simulink model "worldbased"  (R2021a)
settings: Solver=VariableStepAuto  StartTime=0.0  StopTime=60  RelTol=1e-3
libraries: pid_lib x4, mpclib x1, aerolibfltsims x1
settings Model: Creator=ZumoArthicha  LastModifiedBy=ZumoArthicha

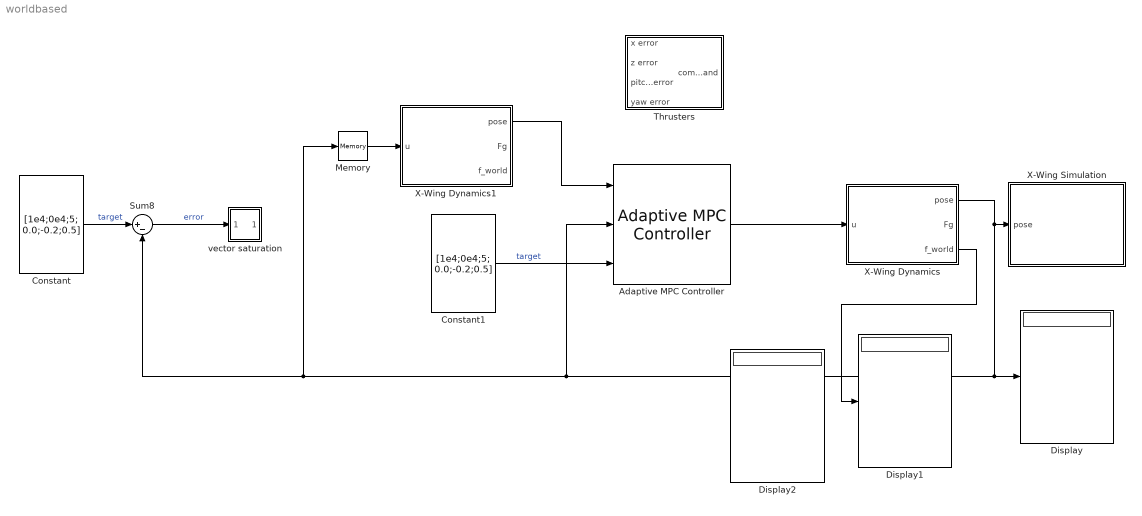
== system worldbased ==
  Adaptive MPC Controller : mpclib/Adaptive MPC Controller  SCDEnableBlockLinearizationSpecification=on  x0=[0;0;0;0;0;0]  enable_value=0  updateMPCinCallerWorkspace=on  md_inport=off  mv_inport=off  uref_inport=off  return_cost=off  return_mvseq=off  return_qpstatus=off  return_xseq=off  return_state=off  return_ovseq=off  state_inport=off  isltv_plant=off  umin_inport=off  umax_inport=off  ymin_inport=off  ymax_inport=off  cc_inport=off  ywt_inport=off  uwt_inport=off  duwt_inport=off  rhoeps_inport=off  pm_inport=off  MaximumP=10  HorizonChoice=FixedHorizon  BlockDataType=double  SampleTimeInherited=off  switch_inport=off
  Constant : Constant  Value=[1e4;0e4;5; 0.0;-0.2;0.5]  VectorParams1D=off
  Constant1 : Constant  Value=[1e4;0e4;5; 0.0;-0.2;0.5]  VectorParams1D=off
  Display : Display
  Display1 : Display
  Display2 : Display
  Memory : Memory
  Sum8 : Sum  Inputs=|+-
  Thrusters : Subsystem
      mask Display: image(imread("pictures/thrusters.PNG"))
  X-Wing Dynamics : Subsystem
      mask Display: image(imread("pictures/simplified_model.png"))
  X-Wing Dynamics1 : Subsystem
      mask Display: image(imread("pictures/simplified_model.png"))
  X-Wing Simulation : Subsystem
      mask Display: image(imread("pictures/simulation.PNG"))
  vector saturation : Subsystem
  wires:
  X-Wing Dynamics/1(pose) -> Display/1, Adaptive MPC Controller/2, Memory/1, Sum8/2, X-Wing Simulation/1(pose)
  Constant/1 -> Sum8/1  "target"
  Sum8/1 -> vector saturation/1(Input)  "error"
  X-Wing Dynamics/3(f_world) -> Display1/1
  Adaptive MPC Controller/1 -> X-Wing Dynamics/1(u)
  Constant1/1 -> Adaptive MPC Controller/3  "target"
  X-Wing Dynamics1/1(pose) -> Adaptive MPC Controller/1
  Memory/1 -> X-Wing Dynamics1/1(u)

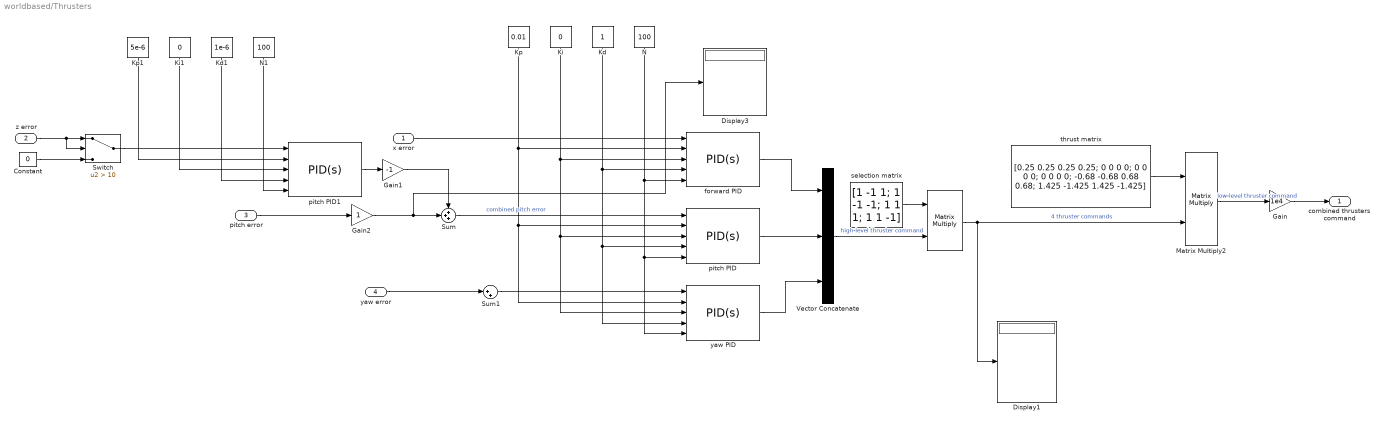
== system worldbased/Thrusters ==
  x error : Inport
  z error : Inport  Port=2
  pitch error : Inport  Port=3
  yaw error : Inport  Port=4
  "  " : Product  Multiplication=Matrix(*)
  Constant : Constant  Value=0
  Display1 : Display
  Display3 : Display
  Gain : Gain  Gain=1e4
  Gain1 : Gain  Gain=-1
  Gain2 : Gain
  Kd : Constant
  Kd1 : Constant  Value=1e-6
  Ki : Constant  Value=0
  Ki1 : Constant  Value=0
  Kp : Constant  Value=0.01
  Kp1 : Constant  Value=5e-6
  Matrix Multiply2 : Product  Multiplication=Matrix(*)
  N : Constant  Value=100
  N1 : Constant  Value=100
  Sum : Sum  Inputs=+++
  Sum1 : Sum  Inputs=|++
  Switch : Switch  Criteria=u2 > Threshold  Threshold=10
  Vector Concatenate : Concatenate  NumInputs=3
  forward PID : pid_lib/PID Controller  Controller=PID  Form=Parallel  TimeDomain=Continuous-time  UseExternalTs=off  SampleTime=-1  IntegratorMethod=Forward Euler  FilterMethod=Forward Euler  ControllerParametersSource=external  P=0.01  I=0  D=1  UseFilter=on  N=100  TunerSelectOption=Transfer Function Based (PID Tuner App)  InitialConditionSource=internal  InitialConditionForIntegrator=0  InitialConditionForFilter=0  DifferentiatorICPrevScaledInput=0  ExternalReset=none  TrackingMode=off  Kt=1  LimitOutput=off  SatLimitsSource=internal  UpperSaturationLimit=inf  LowerSaturationLimit=-inf  LinearizeAsGain=on  AntiWindupMode=none  Kb=1  POutMin=[]  POutMax=[]  IOutMin=[]  IOutMax=[]  DOutMin=[]  DOutMax=[]  NOutMin=[]  NOutMax=[]  SumOutMin=[]  SumOutMax=[]  SaturationOutMin=[]  SaturationOutMax=[]  PParamMin=[]  PParamMax=[]  IParamMin=[]  IParamMax=[]  DParamMin=[]  DParamMax=[]  NParamMin=[]  NParamMax=[]  KbParamMin=[]  KbParamMax=[]  KtParamMin=[]  KtParamMax=[]  KbOutMin=[]  KbOutMax=[]  KtOutMin=[]  KtOutMax=[]  IntegratorOutMin=[]  IntegratorOutMax=[]  FilterOutMin=[]  FilterOutMax=[]  SumI1OutMin=[]  SumI1OutMax=[]  SumI2OutMin=[]  SumI2OutMax=[]  SumI3OutMin=[]  SumI3OutMax=[]  SumI4OutMin=[]  SumI4OutMax=[]  SumDOutMin=[]  SumDOutMax=[]  DifferentiatorOutMin=[]  DifferentiatorOutMax=[]  FilterDiffOutCoefMin=[]  FilterDiffOutCoefMax=[]  ReciprocalOutMin=[]  ReciprocalOutMax=[]  SumDenOutMin=[]  SumDenOutMax=[]  SumNumOutMin=[]  SumNumOutMax=[]  DivideOutMin=[]  DivideOutMax=[]  UdiffTsProdOutMin=[]  UdiffTsProdOutMax=[]  NTsProdOutMin=[]  NTsProdOutMax=[]  UintegralTsProdOutMin=[]  UintegralTsProdOutMax=[]  UngainTsProdOutMin=[]  UngainTsProdOutMax=[]  IntegratorContinuousStateAttributes=''  IntegratorStateMustResolveToSignalObject=off  IntegratorRTWStateStorageClass=Auto  FilterContinuousStateAttributes=''  FilterStateMustResolveToSignalObject=off  FilterRTWStateStorageClass=Auto  ParallelPVariant=ExternalParameters  IdealPVariant=Disabled  IVariant=ExternalParameters  DVariant=ExternalParameters  IntegratorVariant=Continuous  SatVariant=Disabled  AWVariant=Passthrough  PCopyVariant=Disabled  TRVariant=Disabled  FdbkBlocksVariant=Forward  IdealPFdbkVariant=Disabled  SatFdbkVariant=Disabled  DerivativeFilterVariant=ContFilter  NVariant=ExternalParameters  NCopyVariant=Disabled  FilterICVariant=InternalICsFilter  IntegratorICVariant=InternalICs  ExternalResetVariant=Disabled  TRSumVariant=Passthrough  SumFdbkVariant=Disabled  SumVariant=Sum_PID  TsampFilterVariant=InternalTs  TsampNgainVariant=Passthrough  TsampIntegralVariant=Passthrough  ExternalSaturationOutDataTypeStr=Inherit: Same as second input
  pitch PID : pid_lib/PID Controller  Controller=PID  Form=Parallel  TimeDomain=Continuous-time  UseExternalTs=off  SampleTime=-1  IntegratorMethod=Forward Euler  FilterMethod=Forward Euler  ControllerParametersSource=external  P=0.01  I=0  D=1  UseFilter=on  N=100  TunerSelectOption=Transfer Function Based (PID Tuner App)  InitialConditionSource=internal  InitialConditionForIntegrator=0  InitialConditionForFilter=0  DifferentiatorICPrevScaledInput=0  ExternalReset=none  TrackingMode=off  Kt=1  LimitOutput=off  SatLimitsSource=internal  UpperSaturationLimit=inf  LowerSaturationLimit=-inf  LinearizeAsGain=on  AntiWindupMode=none  Kb=1  POutMin=[]  POutMax=[]  IOutMin=[]  IOutMax=[]  DOutMin=[]  DOutMax=[]  NOutMin=[]  NOutMax=[]  SumOutMin=[]  SumOutMax=[]  SaturationOutMin=[]  SaturationOutMax=[]  PParamMin=[]  PParamMax=[]  IParamMin=[]  IParamMax=[]  DParamMin=[]  DParamMax=[]  NParamMin=[]  NParamMax=[]  KbParamMin=[]  KbParamMax=[]  KtParamMin=[]  KtParamMax=[]  KbOutMin=[]  KbOutMax=[]  KtOutMin=[]  KtOutMax=[]  IntegratorOutMin=[]  IntegratorOutMax=[]  FilterOutMin=[]  FilterOutMax=[]  SumI1OutMin=[]  SumI1OutMax=[]  SumI2OutMin=[]  SumI2OutMax=[]  SumI3OutMin=[]  SumI3OutMax=[]  SumI4OutMin=[]  SumI4OutMax=[]  SumDOutMin=[]  SumDOutMax=[]  DifferentiatorOutMin=[]  DifferentiatorOutMax=[]  FilterDiffOutCoefMin=[]  FilterDiffOutCoefMax=[]  ReciprocalOutMin=[]  ReciprocalOutMax=[]  SumDenOutMin=[]  SumDenOutMax=[]  SumNumOutMin=[]  SumNumOutMax=[]  DivideOutMin=[]  DivideOutMax=[]  UdiffTsProdOutMin=[]  UdiffTsProdOutMax=[]  NTsProdOutMin=[]  NTsProdOutMax=[]  UintegralTsProdOutMin=[]  UintegralTsProdOutMax=[]  UngainTsProdOutMin=[]  UngainTsProdOutMax=[]  IntegratorContinuousStateAttributes=''  IntegratorStateMustResolveToSignalObject=off  IntegratorRTWStateStorageClass=Auto  FilterContinuousStateAttributes=''  FilterStateMustResolveToSignalObject=off  FilterRTWStateStorageClass=Auto  ParallelPVariant=ExternalParameters  IdealPVariant=Disabled  IVariant=ExternalParameters  DVariant=ExternalParameters  IntegratorVariant=Continuous  SatVariant=Disabled  AWVariant=Passthrough  PCopyVariant=Disabled  TRVariant=Disabled  FdbkBlocksVariant=Forward  IdealPFdbkVariant=Disabled  SatFdbkVariant=Disabled  DerivativeFilterVariant=ContFilter  NVariant=ExternalParameters  NCopyVariant=Disabled  FilterICVariant=InternalICsFilter  IntegratorICVariant=InternalICs  ExternalResetVariant=Disabled  TRSumVariant=Passthrough  SumFdbkVariant=Disabled  SumVariant=Sum_PID  TsampFilterVariant=InternalTs  TsampNgainVariant=Passthrough  TsampIntegralVariant=Passthrough  ExternalSaturationOutDataTypeStr=Inherit: Same as second input
  pitch PID1 : pid_lib/PID Controller  Controller=PID  Form=Parallel  TimeDomain=Continuous-time  UseExternalTs=off  SampleTime=-1  IntegratorMethod=Forward Euler  FilterMethod=Forward Euler  ControllerParametersSource=external  P=0.01  I=0  D=1  UseFilter=on  N=100  TunerSelectOption=Transfer Function Based (PID Tuner App)  InitialConditionSource=internal  InitialConditionForIntegrator=0  InitialConditionForFilter=0  DifferentiatorICPrevScaledInput=0  ExternalReset=none  TrackingMode=off  Kt=1  LimitOutput=off  SatLimitsSource=internal  UpperSaturationLimit=inf  LowerSaturationLimit=-inf  LinearizeAsGain=on  AntiWindupMode=none  Kb=1  POutMin=[]  POutMax=[]  IOutMin=[]  IOutMax=[]  DOutMin=[]  DOutMax=[]  NOutMin=[]  NOutMax=[]  SumOutMin=[]  SumOutMax=[]  SaturationOutMin=[]  SaturationOutMax=[]  PParamMin=[]  PParamMax=[]  IParamMin=[]  IParamMax=[]  DParamMin=[]  DParamMax=[]  NParamMin=[]  NParamMax=[]  KbParamMin=[]  KbParamMax=[]  KtParamMin=[]  KtParamMax=[]  KbOutMin=[]  KbOutMax=[]  KtOutMin=[]  KtOutMax=[]  IntegratorOutMin=[]  IntegratorOutMax=[]  FilterOutMin=[]  FilterOutMax=[]  SumI1OutMin=[]  SumI1OutMax=[]  SumI2OutMin=[]  SumI2OutMax=[]  SumI3OutMin=[]  SumI3OutMax=[]  SumI4OutMin=[]  SumI4OutMax=[]  SumDOutMin=[]  SumDOutMax=[]  DifferentiatorOutMin=[]  DifferentiatorOutMax=[]  FilterDiffOutCoefMin=[]  FilterDiffOutCoefMax=[]  ReciprocalOutMin=[]  ReciprocalOutMax=[]  SumDenOutMin=[]  SumDenOutMax=[]  SumNumOutMin=[]  SumNumOutMax=[]  DivideOutMin=[]  DivideOutMax=[]  UdiffTsProdOutMin=[]  UdiffTsProdOutMax=[]  NTsProdOutMin=[]  NTsProdOutMax=[]  UintegralTsProdOutMin=[]  UintegralTsProdOutMax=[]  UngainTsProdOutMin=[]  UngainTsProdOutMax=[]  IntegratorContinuousStateAttributes=''  IntegratorStateMustResolveToSignalObject=off  IntegratorRTWStateStorageClass=Auto  FilterContinuousStateAttributes=''  FilterStateMustResolveToSignalObject=off  FilterRTWStateStorageClass=Auto  ParallelPVariant=ExternalParameters  IdealPVariant=Disabled  IVariant=ExternalParameters  DVariant=ExternalParameters  IntegratorVariant=Continuous  SatVariant=Disabled  AWVariant=Passthrough  PCopyVariant=Disabled  TRVariant=Disabled  FdbkBlocksVariant=Forward  IdealPFdbkVariant=Disabled  SatFdbkVariant=Disabled  DerivativeFilterVariant=ContFilter  NVariant=ExternalParameters  NCopyVariant=Disabled  FilterICVariant=InternalICsFilter  IntegratorICVariant=InternalICs  ExternalResetVariant=Disabled  TRSumVariant=Passthrough  SumFdbkVariant=Disabled  SumVariant=Sum_PID  TsampFilterVariant=InternalTs  TsampNgainVariant=Passthrough  TsampIntegralVariant=Passthrough  ExternalSaturationOutDataTypeStr=Inherit: Same as second input
  selection matrix : Constant  Value=[1 -1 1; 1 -1 -1; 1 1 1; 1 1 -1]  VectorParams1D=off
  thrust matrix : Constant  Value=[0.25 0.25 0.25 0.25; 0 0 0 0; 0 0 0 0; 0 0 0 0; -0.68 -0.68 0.68 0.68; 1.425 -1.425 1.425 -1.425]  VectorParams1D=off
  yaw PID : pid_lib/PID Controller  Controller=PID  Form=Parallel  TimeDomain=Continuous-time  UseExternalTs=off  SampleTime=-1  IntegratorMethod=Forward Euler  FilterMethod=Forward Euler  ControllerParametersSource=external  P=0.01  I=0  D=1  UseFilter=on  N=100  TunerSelectOption=Transfer Function Based (PID Tuner App)  InitialConditionSource=internal  InitialConditionForIntegrator=0  InitialConditionForFilter=0  DifferentiatorICPrevScaledInput=0  ExternalReset=none  TrackingMode=off  Kt=1  LimitOutput=off  SatLimitsSource=internal  UpperSaturationLimit=inf  LowerSaturationLimit=-inf  LinearizeAsGain=on  AntiWindupMode=none  Kb=1  POutMin=[]  POutMax=[]  IOutMin=[]  IOutMax=[]  DOutMin=[]  DOutMax=[]  NOutMin=[]  NOutMax=[]  SumOutMin=[]  SumOutMax=[]  SaturationOutMin=[]  SaturationOutMax=[]  PParamMin=[]  PParamMax=[]  IParamMin=[]  IParamMax=[]  DParamMin=[]  DParamMax=[]  NParamMin=[]  NParamMax=[]  KbParamMin=[]  KbParamMax=[]  KtParamMin=[]  KtParamMax=[]  KbOutMin=[]  KbOutMax=[]  KtOutMin=[]  KtOutMax=[]  IntegratorOutMin=[]  IntegratorOutMax=[]  FilterOutMin=[]  FilterOutMax=[]  SumI1OutMin=[]  SumI1OutMax=[]  SumI2OutMin=[]  SumI2OutMax=[]  SumI3OutMin=[]  SumI3OutMax=[]  SumI4OutMin=[]  SumI4OutMax=[]  SumDOutMin=[]  SumDOutMax=[]  DifferentiatorOutMin=[]  DifferentiatorOutMax=[]  FilterDiffOutCoefMin=[]  FilterDiffOutCoefMax=[]  ReciprocalOutMin=[]  ReciprocalOutMax=[]  SumDenOutMin=[]  SumDenOutMax=[]  SumNumOutMin=[]  SumNumOutMax=[]  DivideOutMin=[]  DivideOutMax=[]  UdiffTsProdOutMin=[]  UdiffTsProdOutMax=[]  NTsProdOutMin=[]  NTsProdOutMax=[]  UintegralTsProdOutMin=[]  UintegralTsProdOutMax=[]  UngainTsProdOutMin=[]  UngainTsProdOutMax=[]  IntegratorContinuousStateAttributes=''  IntegratorStateMustResolveToSignalObject=off  IntegratorRTWStateStorageClass=Auto  FilterContinuousStateAttributes=''  FilterStateMustResolveToSignalObject=off  FilterRTWStateStorageClass=Auto  ParallelPVariant=ExternalParameters  IdealPVariant=Disabled  IVariant=ExternalParameters  DVariant=ExternalParameters  IntegratorVariant=Continuous  SatVariant=Disabled  AWVariant=Passthrough  PCopyVariant=Disabled  TRVariant=Disabled  FdbkBlocksVariant=Forward  IdealPFdbkVariant=Disabled  SatFdbkVariant=Disabled  DerivativeFilterVariant=ContFilter  NVariant=ExternalParameters  NCopyVariant=Disabled  FilterICVariant=InternalICsFilter  IntegratorICVariant=InternalICs  ExternalResetVariant=Disabled  TRSumVariant=Passthrough  SumFdbkVariant=Disabled  SumVariant=Sum_PID  TsampFilterVariant=InternalTs  TsampNgainVariant=Passthrough  TsampIntegralVariant=Passthrough  ExternalSaturationOutDataTypeStr=Inherit: Same as second input
  combined thrusters command : Outport  PortDimensions=6
  wires:
  N/1 -> yaw PID/5, pitch PID/5, forward PID/5
  Kd/1 -> pitch PID/4, yaw PID/4, forward PID/4
  Ki/1 -> yaw PID/3, pitch PID/3, forward PID/3
  Kp/1 -> pitch PID/2, yaw PID/2, forward PID/2
  yaw PID/1 -> Vector Concatenate/3
  x error/1 -> forward PID/1
  selection matrix/1 -> "  "/1
  Gain/1 -> combined thrusters command/1
  Matrix Multiply2/1 -> Gain/1  "low-level thruster command"
  thrust matrix/1 -> Matrix Multiply2/1
  Vector Concatenate/1 -> "  "/2  "high-level thruster command"
  "  "/1 -> Display1/1, Matrix Multiply2/2  "4 thruster commands"
  pitch PID1/1 -> Gain1/1
  Kp1/1 -> pitch PID1/2
  Ki1/1 -> pitch PID1/3
  Kd1/1 -> pitch PID1/4
  N1/1 -> pitch PID1/5
  Constant/1 -> Switch/3
  Switch/1 -> pitch PID1/1
  Sum/1 -> pitch PID/1  "combined pitch error"
  z error/1 -> Switch/2, Switch/1
  Gain2/1 -> Display3/1, Sum/2
  Sum1/1 -> yaw PID/1
  pitch PID/1 -> Vector Concatenate/2
  forward PID/1 -> Vector Concatenate/1
  pitch error/1 -> Gain2/1
  Gain1/1 -> Sum/1
  yaw error/1 -> Sum1/1

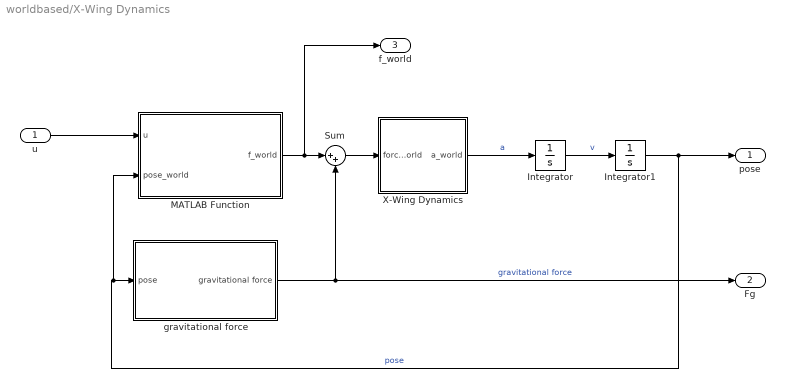
== system worldbased/X-Wing Dynamics ==
  u : Inport
  Integrator : Integrator  InitialCondition=[0;0;0;0;0;0]
  Integrator1 : Integrator  InitialCondition=[0;0;0;0;0;0]
  MATLAB Function : MATLAB Function  TreatAsAtomicUnit=on
  Sum : Sum  Inputs=|++
  X-Wing Dynamics : MATLAB Function  TreatAsAtomicUnit=on
  gravitational force : Subsystem
      mask Display: image(imread("pictures/gravitational_force.PNG"))
  pose : Outport
  Fg : Outport  Port=2
  f_world : Outport  Port=3
  wires:
  gravitational force/1(gravitational force) -> Fg/1, Sum/2  "gravitational force"
  Integrator/1 -> Integrator1/1  "v"
  Sum/1 -> X-Wing Dynamics/1(force_world)
  X-Wing Dynamics/1(a_world) -> Integrator/1  "a"
  Integrator1/1 -> pose/1, MATLAB Function/2(pose_world), gravitational force/1(pose)  "pose"
  u/1 -> MATLAB Function/1(u)
  MATLAB Function/1(f_world) -> f_world/1, Sum/1

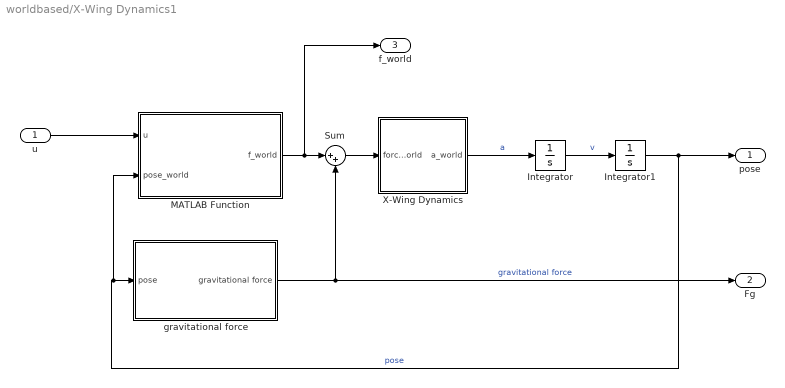
== system worldbased/X-Wing Dynamics1 ==
  u : Inport
  Integrator : Integrator  InitialCondition=[0;0;0;0;0;0]
  Integrator1 : Integrator  InitialCondition=[0;0;0;0;0;0]
  MATLAB Function : MATLAB Function  TreatAsAtomicUnit=on
  Sum : Sum  Inputs=|++
  X-Wing Dynamics : MATLAB Function  TreatAsAtomicUnit=on
  gravitational force : Subsystem
      mask Display: image(imread("pictures/gravitational_force.PNG"))
  pose : Outport
  Fg : Outport  Port=2
  f_world : Outport  Port=3
  wires:
  gravitational force/1(gravitational force) -> Fg/1, Sum/2  "gravitational force"
  Integrator/1 -> Integrator1/1  "v"
  Sum/1 -> X-Wing Dynamics/1(force_world)
  X-Wing Dynamics/1(a_world) -> Integrator/1  "a"
  Integrator1/1 -> pose/1, MATLAB Function/2(pose_world), gravitational force/1(pose)  "pose"
  u/1 -> MATLAB Function/1(u)
  MATLAB Function/1(f_world) -> f_world/1, Sum/1

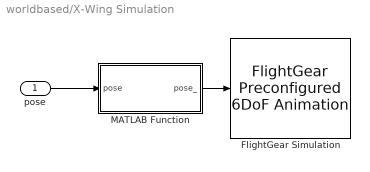
== system worldbased/X-Wing Simulation ==
  pose : Inport
  FlightGear Simulation : aerolibfltsims/FlightGear Preconfigured 6DoF Animation  xFlightGearVersion=v2019.1  DestinationIpAddress=127.0.0.1  DestinationPort=5502  SampleTime=1/30  packetVersion=24  mask(FlightGearQuick6DoFAnimation){}
      mask Display:
      | % This is a new mask on top of the base mask.
      | % Use "View base mask" link below to see the base mask.
      | image(imread("pictures/simulation.PNG"))
  MATLAB Function : MATLAB Function  TreatAsAtomicUnit=on
  wires:
  MATLAB Function/1(pose_) -> FlightGear Simulation/1
  pose/1 -> MATLAB Function/1(pose)

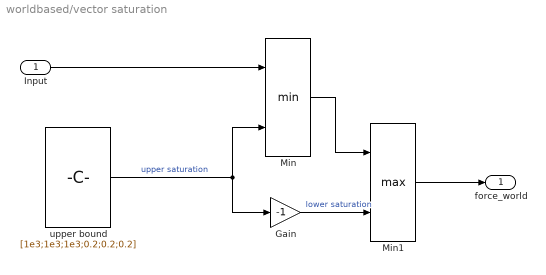
== system worldbased/vector saturation ==
  Input : Inport
  Gain : Gain  Gain=-1
  Min : MinMax  Inputs=2
  Min1 : MinMax  Function=max  Inputs=2
  upper bound : Constant  Value=[1e3;1e3;1e3;0.2;0.2;0.2]  VectorParams1D=off
  force_world : Outport
  wires:
  Input/1 -> Min/1
  upper bound/1 -> Min/2, Gain/1  "upper saturation"
  Min/1 -> Min1/1
  Gain/1 -> Min1/2  "lower saturation"
  Min1/1 -> force_world/1

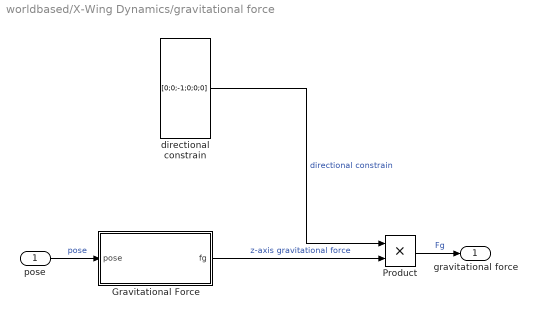
== system worldbased/X-Wing Dynamics/gravitational force ==
  pose : Inport
  Gravitational Force : MATLAB Function  TreatAsAtomicUnit=on
  Product : Product
  directional constrain : Constant  Value=[0;0;-1;0;0;0]  VectorParams1D=off
  gravitational force : Outport  PortDimensions=6
  wires:
  directional constrain/1 -> Product/1  "directional constrain"
  Gravitational Force/1(fg) -> Product/2  "z-axis gravitational force"
  pose/1 -> Gravitational Force/1(pose)  "pose"
  Product/1 -> gravitational force/1  "Fg"

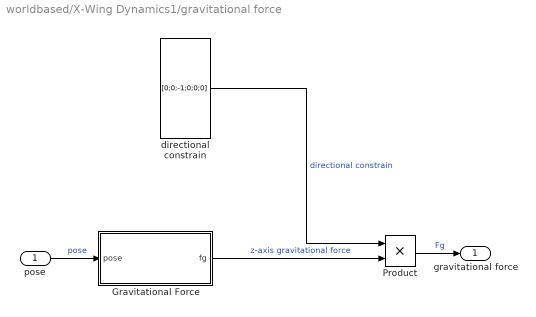
== system worldbased/X-Wing Dynamics1/gravitational force ==
  pose : Inport
  Gravitational Force : MATLAB Function  TreatAsAtomicUnit=on
  Product : Product
  directional constrain : Constant  Value=[0;0;-1;0;0;0]  VectorParams1D=off
  gravitational force : Outport  PortDimensions=6
  wires:
  directional constrain/1 -> Product/1  "directional constrain"
  Gravitational Force/1(fg) -> Product/2  "z-axis gravitational force"
  pose/1 -> Gravitational Force/1(pose)  "pose"
  Product/1 -> gravitational force/1  "Fg"

== matlab function worldbased/X-Wing Dynamics1/X-Wing Dynamics ==
  data: force_world input; a_world output
function a_world = fcn(force_world)

% force_world = [fx; fy; fz; mx; my; mz];

% define the parameters
% inertia and mass
I = [36145 0 0; 2.26927 116437.915354 0.00035374516; 0 0.00035374516 90590.2796914]; % innertia matrix
m = 10000;
a_world = [(1/m)*diag([1 1 1]) zeros(3,3); zeros(3,3) inv(I)]*force_world;

== matlab function worldbased/X-Wing Dynamics1/gravitational force/Gravitational Force ==
  data: pose input; fg output
function fg = gravitational_force(pose)


G = 6.67259*10^-11; % gravitational constant < Nm2/kg2 >
M = 5.98*10^24; % earth mass <kg>
R = 6.38*10^6; % average earth radius <m>
r = R + pose(3); % distance from the surface <m>
m = 10000; % X-Wing mass <kg>
fg = G*m*M/(r*r); % F = Gmm/r^2

end

== matlab function worldbased/X-Wing Dynamics/X-Wing Dynamics ==
  data: force_world input; a_world output
function a_world = fcn(force_world)

% force_world = [fx; fy; fz; mx; my; mz];

% define the parameters
% inertia and mass
I = [36145 0 0; 2.26927 116437.915354 0.00035374516; 0 0.00035374516 90590.2796914]; % innertia matrix
m = 10000;
a_world = [(1/m)*diag([1 1 1]) zeros(3,3); zeros(3,3) inv(I)]*force_world;

== matlab function worldbased/X-Wing Dynamics/MATLAB Function ==
  data: u input; f_world output; pose_world input
function f_world = actuator_force(u,pose_world)

% force transofrmation matrix w.r.t body
T = [1 1 1 1 0 0;
    0 0 0 0 0 0;
    0 0 0 0 1 0;
    0 0 0 0 0 1;
    0.68 0.68 -0.68 -0.68 0 0;
    -1.425 1.425 -1.425 1.425 0 0;];



% compute force w.r.t. body
f_body = T*u;

% compute force w.r.t. world
R = rotz(rad2deg(pose_world(6)))*roty(rad2deg(pose_world(5)))*rotx(rad2deg(pose_world(4)));
f_world = [R*f_body(1:3);f_body(4:6)]; % force w.r.t. world

end

== matlab function worldbased/X-Wing Simulation/MATLAB Function ==
  data: pose input; pose_ output
function pose_ = simulation_interface(pose)
R = 6.38*10^6; % average earth radius <m>
x = -100*pose(1)/R; % flip the x-axis;
y = 100*pose(2)/R;
z = pose(3);

position = [x;y;z]+[-45;83.1;0];
pose_ = [position;-pose(5);-pose(4);pose(6)];
end

== matlab function worldbased/X-Wing Dynamics/gravitational force/Gravitational Force ==
  data: pose input; fg output
function fg = gravitational_force(pose)


G = 6.67259*10^-11; % gravitational constant < Nm2/kg2 >
M = 5.98*10^24; % earth mass <kg>
R = 6.38*10^6; % average earth radius <m>
r = R + pose(3); % distance from the surface <m>
m = 10000; % X-Wing mass <kg>
fg = G*m*M/(r*r); % F = Gmm/r^2

end

== matlab function worldbased/X-Wing Dynamics1/MATLAB Function ==
  data: u input; f_world output; pose_world input
function f_world = actuator_force(u,pose_world)

% force transofrmation matrix w.r.t body
T = [1 1 1 1 0 0;
    0 0 0 0 0 0;
    0 0 0 0 1 0;
    0 0 0 0 0 1;
    0.68 0.68 -0.68 -0.68 0 0;
    -1.425 1.425 -1.425 1.425 0 0;];



% compute force w.r.t. body
f_body = T*u;

% compute force w.r.t. world
R = rotz(rad2deg(pose_world(6)))*roty(rad2deg(pose_world(5)))*rotx(rad2deg(pose_world(4)));
f_world = [R*f_body(1:3);f_body(4:6)]; % force w.r.t. world

end
